simulink model "p3"  (R2024b)
settings: Solver=ode45  StartTime=0.0  StopTime=30000  MaxStep=0.24  RelTol=1e-3
libraries: fuzblock x1
settings Model: Creator=Borjazz  LastModifiedBy=Borjazz

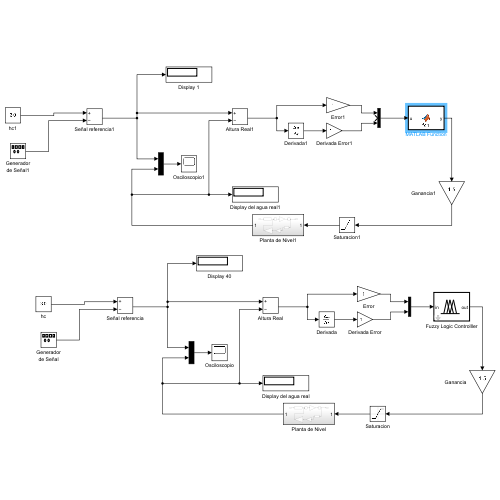
[thumbnail: Simulink's stored preview of the top-level diagram]
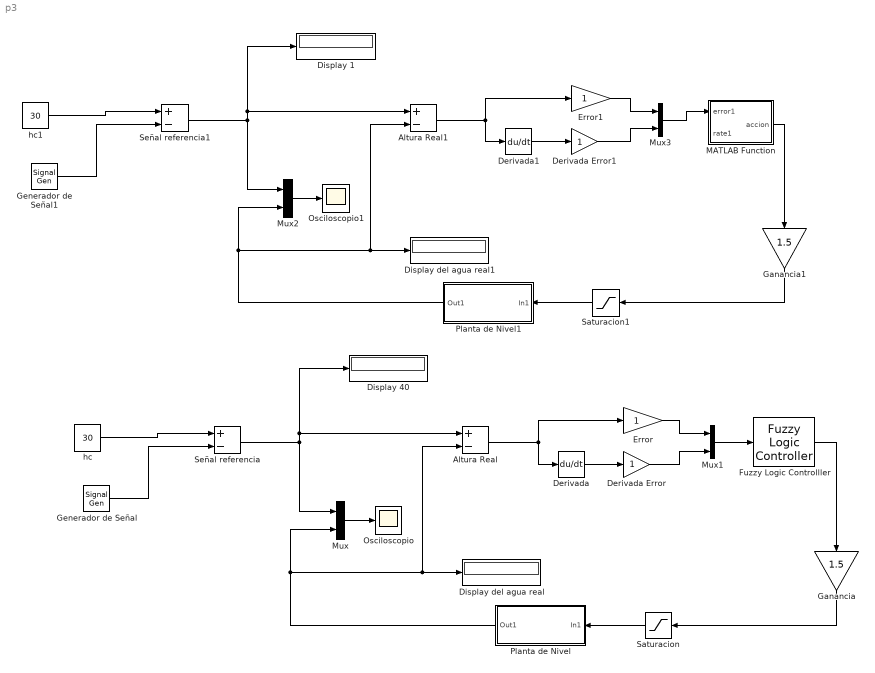
== system p3 ==
  Altura Real : Sum  Inputs=+-
  Altura Real1 : Sum  Inputs=+-
  Derivada : Derivative
  Derivada Error : Gain
  Derivada Error1 : Gain
  Derivada1 : Derivative
  Display 1 : Display
  Display 40 : Display
  Display del agua real : Display
  Display del agua real1 : Display
  Error : Gain
  Error1 : Gain
  Fuzzy Logic Controlller : fuzblock/Fuzzy Logic  Controller  FIS='Practica1.fis'  OutputSampleNumber=101  DataType=double  FuzzifiedInputs=off  RuleFiringStrengths=off  RuleOutputs=off  AggregatedOutputs=off  SimulateUsing=Interpreted execution  OutOfRangeInputValueMessage=warning  NoRuleFiredMessage=warning  EmptyOutputFuzzySetMessage=warning
  Ganancia : Gain  Gain=1.5
  Ganancia1 : Gain  Gain=1.5
  Generador de Señal : SignalGenerator  Amplitude=10  Frequency=0.0125  Units=rad/sec
  Generador de Señal1 : SignalGenerator  Amplitude=10  Frequency=0.0125  Units=rad/sec
  MATLAB Function : MATLAB Function  TreatAsAtomicUnit=on
  Mux : Mux  Inputs=2
  Mux1 : Mux  Inputs=2
  Mux2 : Mux  Inputs=2
  Mux3 : Mux  Inputs=3
  Osciloscopio : Scope
  Osciloscopio1 : Scope
  Planta de Nivel : Subsystem
  Planta de Nivel1 : Subsystem
  Saturacion : Saturate  UpperLimit=1  LowerLimit=0  LinearizeAsGain=off
  Saturacion1 : Saturate  UpperLimit=1  LowerLimit=0  LinearizeAsGain=off
  Señal referencia : Sum  Inputs=+-
  Señal referencia1 : Sum  Inputs=+-
  hc : Constant  Value=30
  hc1 : Constant  Value=30
  wires:
  Ganancia/1 -> Saturacion/1
  Fuzzy Logic Controlller/1 -> Ganancia/1
  Mux1/1 -> Fuzzy Logic Controlller/1
  Error/1 -> Mux1/1
  Derivada Error/1 -> Mux1/2
  Derivada/1 -> Derivada Error/1
  Altura Real/1 -> Error/1, Derivada/1
  Generador de Señal/1 -> Señal referencia/2
  hc/1 -> Señal referencia/1
  Señal referencia/1 -> Altura Real/1, Display 40/1, Mux/1
  Mux/1 -> Osciloscopio/1
  Planta de Nivel/1(Out1) -> Altura Real/2, Display del agua real/1, Mux/2
  Saturacion/1 -> Planta de Nivel/1(In1)
  Saturacion1/1 -> Planta de Nivel1/1(In1)
  Error1/1 -> Mux3/1
  Señal referencia1/1 -> Altura Real1/1, Display 1/1, Mux2/1
  Derivada Error1/1 -> Mux3/3
  hc1/1 -> Señal referencia1/1
  MATLAB Function/1(accion) -> Ganancia1/1
  Planta de Nivel1/1(Out1) -> Altura Real1/2, Display del agua real1/1, Mux2/2
  Mux2/1 -> Osciloscopio1/1
  Mux3/1 -> MATLAB Function/1(error1)
  Derivada1/1 -> Derivada Error1/1
  Generador de Señal1/1 -> Señal referencia1/2
  Altura Real1/1 -> Error1/1, Derivada1/1
  Ganancia1/1 -> Saturacion1/1

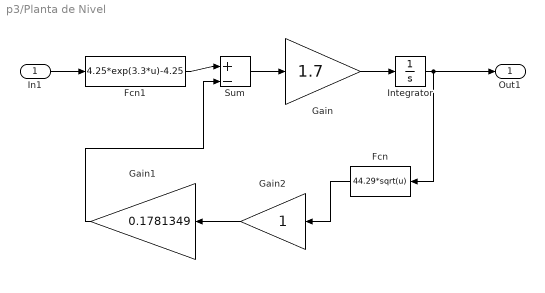
== system p3/Planta de Nivel ==
  In1 : Inport
  Fcn : Fcn  Expr=44.29*sqrt(u)
  Fcn1 : Fcn  Expr=4.25*exp(3.3*u)-4.25
  Gain : Gain  Gain=1.7
  Gain1 : Gain  Gain=0.1781349
  Gain2 : Gain
  Integrator : Integrator  InitialCondition=15  LimitOutput=on  UpperSaturationLimit=40  LowerSaturationLimit=20
  Sum : Sum  Inputs=|+-
  Out1 : Outport
  wires:
  Integrator/1 -> Fcn/1, Out1/1
  Gain2/1 -> Gain1/1
  Gain/1 -> Integrator/1
  Gain1/1 -> Sum/2
  Fcn1/1 -> Sum/1
  Sum/1 -> Gain/1
  In1/1 -> Fcn1/1
  Fcn/1 -> Gain2/1

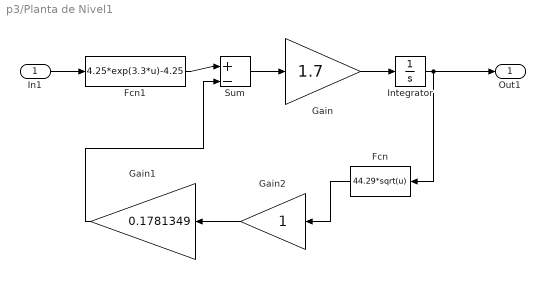
== system p3/Planta de Nivel1 ==
  In1 : Inport
  Fcn : Fcn  Expr=44.29*sqrt(u)
  Fcn1 : Fcn  Expr=4.25*exp(3.3*u)-4.25
  Gain : Gain  Gain=1.7
  Gain1 : Gain  Gain=0.1781349
  Gain2 : Gain
  Integrator : Integrator  InitialCondition=15  LimitOutput=on  UpperSaturationLimit=40  LowerSaturationLimit=20
  Sum : Sum  Inputs=|+-
  Out1 : Outport
  wires:
  Integrator/1 -> Fcn/1, Out1/1
  Gain2/1 -> Gain1/1
  Gain/1 -> Integrator/1
  Gain1/1 -> Sum/2
  Fcn1/1 -> Sum/1
  Sum/1 -> Gain/1
  In1/1 -> Fcn1/1
  Fcn/1 -> Gain2/1

== matlab function p3/MATLAB Function ==
  data: error1 input; accion output; rate1 input
function accion = CFuzzymin(error1, rate1)
% CFuzzymin - Controlador difuso mínimo
% Entradas:
%   error1: Error de entrada (escalar)
%   rate1: Derivada del error (escalar)
% Salida:
%   accion: Señal de salida del controlador

% Validar que las entradas sean escalares
error1 = error1(1);
rate1 = rate1(1);

% Declaración de constantes
L = 100;
H = 100;
Ge = 2000;
Gr = 1;

% Escalar las señales de entrada
e = Ge * error1;
r = Gr * rate1;

% Inicializar región
ic = 0;

% Región I: e >= 0, r >= 0
if r >= 0 && e >= 0
    if e < L && r >= L
        ic = 11;
    elseif e >= L && r >= L
        ic = 17;
    elseif e < r && e < L
        ic = 3;
    elseif e >= r && e < L
        ic = 2;
    else
        ic = 10;
    end

% Región II: e >= 0, r < 0
elseif r < 0 && e >= 0
    if e > -r && e < L && r > -L
        ic = 1;
    elseif e <= -r && e < L && r > -L
        ic = 8;
    elseif e >= L && r > -L
        ic = 9;
    elseif e < L && r <= -L
        ic = 16;
    else
        ic = 20;
    end

% Región III: e < 0, r >= 0
elseif r >= 0 && e < 0
    if e > -L && r >= L
        ic = 12;
    elseif e <= -L && r >= L
        ic = 18;
    elseif -e <= r && e > -L && r < L
        ic = 4;
    elseif -e > r && e > -L && r < L
        ic = 5;
    else
        ic = 13;
    end

% Región IV: e < 0, r < 0
else
    if -e > -r && e > -L && r > -L
        ic = 6;
    elseif -e < -r && e > -L && r > -L
        ic = 7;
    elseif e <= -L && r > -L
        ic = 14;
    elseif e <= -L && r <= -L
        ic = 19;
    else
        ic = 15;
    end
end

% Selección de acción según región IC
switch ic
    case {1, 2, 5, 6}
        accion = (L * (Ge * error1 + Gr * rate1)) / (2 * (2 * L - (Ge * abs(error1))));
    case {3, 4, 7, 8}
        accion = (L * (Ge * error1 + Gr * rate1)) / (2 * (2 * L - (Gr * abs(rate1))));
    case {9, 10}
        accion = (L + Gr * rate1) / 2;
    case {11, 12}
        accion = (L + Ge * error1) / 2;
    case {13, 14}
        accion = (-L + Gr * rate1) / 2;
    case {15, 16}
        accion = (-L + Ge * error1) / 2;
    case 17
        accion = L;
    case 19
        accion = -L;
    otherwise % casos 18 y 20
        accion = 0;
end
end
